simulink model "quad_angle_mode"  (R2025a)
settings: Solver=VariableStepAuto  StartTime=0.0  StopTime=10.0  RelTol=1e-3
settings Model: Creator=pvsha  LastModifiedBy=nasim

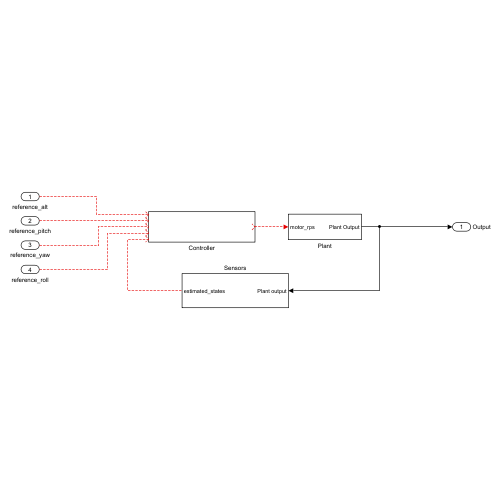
[thumbnail: Simulink's stored preview of the top-level diagram]
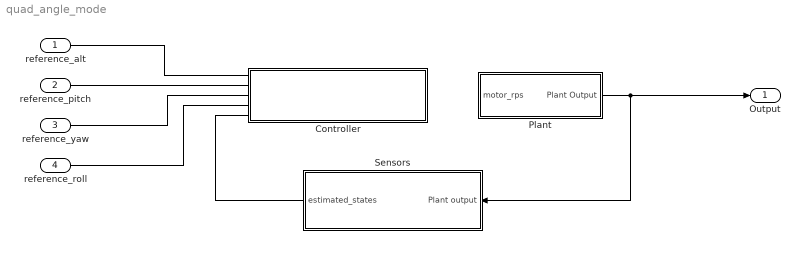
== system quad_angle_mode ==
  reference_alt : Inport
  reference_pitch : Inport  Port=2
  reference_yaw : Inport  Port=3
  reference_roll : Inport  Port=4
  Controller : Subsystem
  Plant : Subsystem
  Sensors : Subsystem
  Output : Outport  SignalName=Output
  wires:
  ? -> Plant/1(motor_rps)
  Sensors/1(estimated_states) -> ?
  Plant/1(Plant Output) -> Sensors/1(Plant output), Output/1
  reference_alt/1 -> ?
  reference_pitch/1 -> ?
  reference_yaw/1 -> ?
  reference_roll/1 -> ?

== system quad_angle_mode/Controller ==

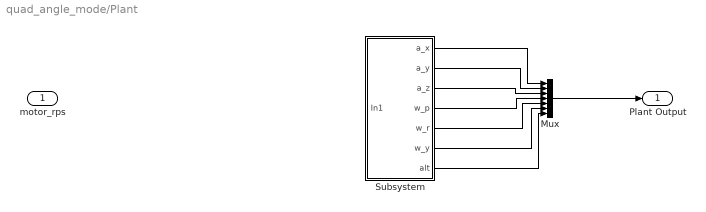
== system quad_angle_mode/Plant ==
  motor_rps : Inport
  Mux : Mux  Inputs=7
  Subsystem : Subsystem
  Plant Output : Outport
  wires:
  Mux/1 -> Plant Output/1
  Subsystem/1(a_x) -> Mux/1
  Subsystem/2(a_y) -> Mux/2
  Subsystem/3(a_z) -> Mux/3
  Subsystem/4(w_p) -> Mux/4
  Subsystem/5(w_r) -> Mux/5
  Subsystem/6(w_y) -> Mux/6
  Subsystem/7(alt) -> Mux/7

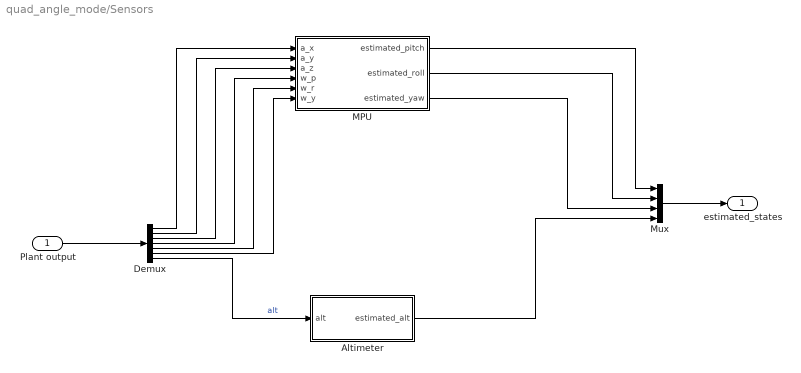
== system quad_angle_mode/Sensors ==
  Plant output : Inport
  Altimeter : Subsystem
  Demux : Demux  Outputs=7
  MPU : Subsystem
  Mux : Mux
  estimated_states : Outport
  wires:
  Plant output/1 -> Demux/1
  Demux/7 -> Altimeter/1(alt)  "alt"
  MPU/2(estimated_roll) -> Mux/2
  MPU/3(estimated_yaw) -> Mux/3
  MPU/1(estimated_pitch) -> Mux/1
  Demux/1 -> MPU/1(a_x)
  Demux/3 -> MPU/3(a_z)
  Demux/2 -> MPU/2(a_y)
  Demux/4 -> MPU/4(w_p)
  Demux/5 -> MPU/5(w_r)
  Demux/6 -> MPU/6(w_y)
  Mux/1 -> estimated_states/1
  Altimeter/1(estimated_alt) -> Mux/4

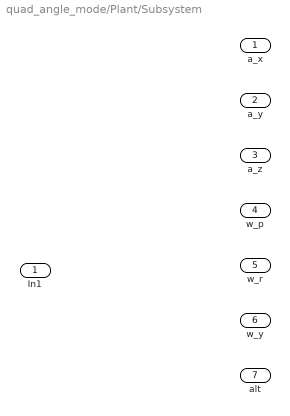
== system quad_angle_mode/Plant/Subsystem ==
  In1 : Inport
  a_x : Outport
  a_y : Outport  Port=2
  a_z : Outport  Port=3
  w_p : Outport  Port=4
  w_r : Outport  Port=5
  w_y : Outport  Port=6
  alt : Outport  Port=7

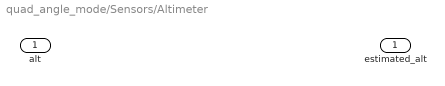
== system quad_angle_mode/Sensors/Altimeter ==
  alt : Inport
  estimated_alt : Outport

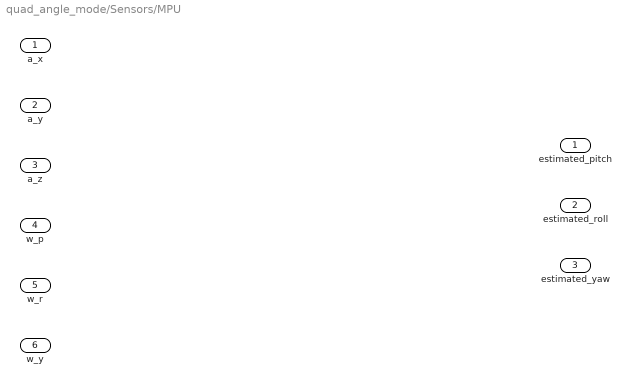
== system quad_angle_mode/Sensors/MPU ==
  a_x : Inport
  a_y : Inport  Port=2
  a_z : Inport  Port=3
  w_p : Inport  Port=4
  w_r : Inport  Port=5
  w_y : Inport  Port=6
  estimated_pitch : Outport
  estimated_roll : Outport  Port=2
  estimated_yaw : Outport  Port=3
